simulink model "MPC_SSM_CurvePathTracking"  (Simulink 8.2)
settings: Solver=ode45  StartTime=0.0  StopTime=400  FixedStep=0.01  RelTol=1e-3
libraries: Solver_SF x1
settings Model: Creator=xuwei  LastModifiedBy=leoking99

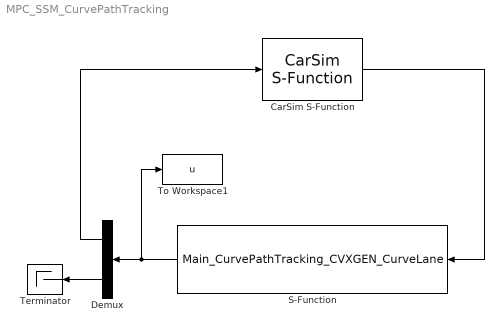
== system MPC_SSM_CurvePathTracking ==
  CarSim S-Function : Solver_SF/CarSim S-Function  Priority=1  VehicleCode=i_s  SIMFILE=LEO_MPC_EM_PathTrackingCtrl.sim
  Demux : Demux  Outputs=[1 7]
  S-Function : S-Function  FunctionName=Main_CurvePathTracking_CVXGEN_CurveLane  EnableBusSupport=off
  Terminator : Terminator
  To Workspace1 : ToWorkspace  VariableName=u  SampleTime=-1  SaveFormat=Structure
  wires:
  CarSim S-Function/1 -> S-Function/1
  S-Function/1 -> Demux/1, To Workspace1/1
  Demux/2 -> Terminator/1
  Demux/1 -> CarSim S-Function/1
